simulink model "Simulation_Rotate_90"  (R2021a)
settings: Solver=FixedStepDiscrete  StartTime=0.0  StopTime=10.0  FixedStep=0.01  RelTol=1e-3
undefined symbols (not defined in the file): axleLength, InputPWM, ticksPerRot, wheelR, WheelSpeed
libraries: mobileRoboticsTrainingLib x5
settings Model: EnablePacing=on  Creator=Boitumelo  LastModifiedBy=akhil

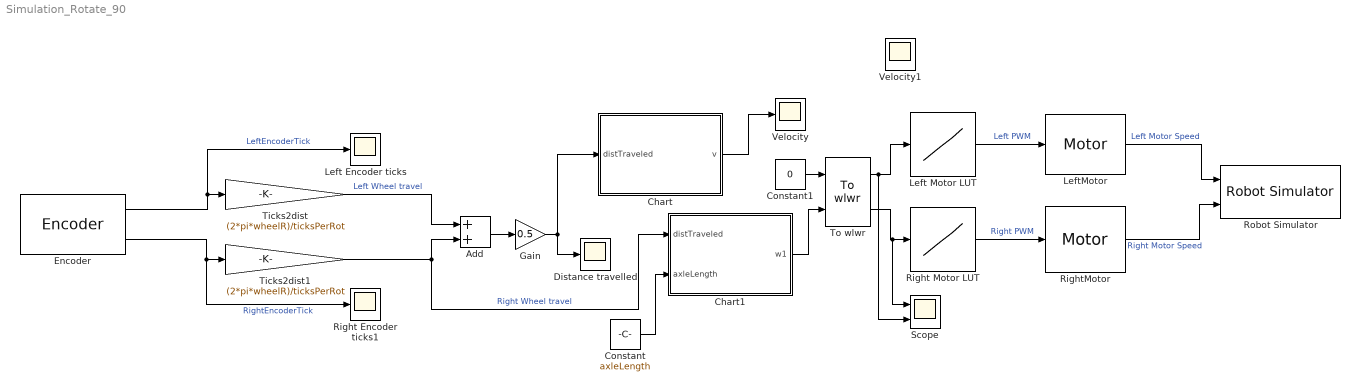
== system Simulation_Rotate_90 ==
  Add : Sum
  Chart : Stateflow chart  TreatAsAtomicUnit=on
  Chart1 : Stateflow chart  TreatAsAtomicUnit=on
  Constant : Constant  Value=axleLength
  Constant1 : Constant  Value=0
  Distance travelled : Scope
  Encoder : mobileRoboticsTrainingLib/Encoder  axleLength=axleLength  wheelR=wheelR  ticksPerRot=ticksPerRot
      settings: SourceProductName=Mobile Robotics Training Library
  Gain : Gain  Gain=0.5
  Left Encoder ticks : Scope
  Left Motor LUT : Lookup_n-D  NumberOfTableDimensions=1  BreakpointsForDimension1=WheelSpeed  Table=InputPWM  InterpMethod=Nearest  ExtrapMethod=Clip  InternalRulePriority=Speed  RndMeth=Simplest  InputSameDT=on
  LeftMotor : mobileRoboticsTrainingLib/Motor  motorPlant=wheelMotorModel  sensorType=Speed
      settings: SourceProductName=Mobile Robotics Training Library
  Right Encoder ticks1 : Scope
  Right Motor LUT : Lookup_n-D  NumberOfTableDimensions=1  BreakpointsForDimension1=WheelSpeed  Table=InputPWM  InterpMethod=Nearest  ExtrapMethod=Clip  InternalRulePriority=Speed  RndMeth=Simplest  InputSameDT=on
  RightMotor : mobileRoboticsTrainingLib/Motor  motorPlant=wheelMotorModel  sensorType=Speed
      settings: SourceProductName=Mobile Robotics Training Library
  Robot Simulator : mobileRoboticsTrainingLib/Robot Simulator  Priority=99  mapVar=[]  startX=1  startY=1  startTheta=0  axleLength=axleLength  wheelR=wheelR
  Scope : Scope  NumInputPorts=2
  Ticks2dist : Gain  Gain=(2*pi*wheelR)/ticksPerRot
  Ticks2dist1 : Gain  Gain=(2*pi*wheelR)/ticksPerRot
  To wlwr : mobileRoboticsTrainingLib/To wlwr  axleLength=0.1  wheelR=0.05
  Velocity : Scope
  Velocity1 : Scope
  wires:
  LeftMotor/1 -> Robot Simulator/1  "Left Motor Speed"
  RightMotor/1 -> Robot Simulator/2  "Right Motor Speed"
  Right Motor LUT/1 -> RightMotor/1  "Right PWM"
  Left Motor LUT/1 -> LeftMotor/1  "Left PWM"
  Encoder/1 -> Left Encoder ticks/1, Ticks2dist/1  "LeftEncoderTick"
  Encoder/2 -> Right Encoder ticks1/1, Ticks2dist1/1  "RightEncoderTick"
  Add/1 -> Gain/1
  Ticks2dist1/1 -> Chart1/1(distTraveled), Add/2  "Right Wheel travel"
  Chart/1(v) -> Velocity/1
  Gain/1 -> Chart/1(distTraveled), Distance travelled/1
  Ticks2dist/1 -> Add/1  "Left Wheel travel"
  Constant/1 -> Chart1/2(axleLength)
  Chart1/1(w1) -> To wlwr/2
  To wlwr/1 -> Scope/2, Left Motor LUT/1
  To wlwr/2 -> Scope/1, Right Motor LUT/1
  Constant1/1 -> To wlwr/1

== stateflow chart Simulation_Rotate_90/Chart1 ==
  state For 90°: pi/2 [commented out]
    For 180°: pi
    for 270°: 3*pi/2
    For 360°: 2*pi
  state Rotate
    entry:
    w1=pi/6
    %wl = -0.55
    %wr = 0.55
  state Stop
    entry:
    w1=0
    %wl = 0
    %wr = 0
  (default) -> Rotate : % Start
  Rotate -> Stop : [2*distTraveled/axleLength >= pi/2]
  Stop -> Rotate : [2*distTraveled/axleLength < pi/2]
  data: distTraveled input; axleLength input; w1 output

== stateflow chart Simulation_Rotate_90/Chart ==
  state MoveForward
    entry:
    v = 0.1
  state Stop
    entry:
    v = 0
  (default) -> MoveForward : % Start
  MoveForward -> Stop : [distTraveled >= 1]
  data: distTraveled input; v output
